simulink model "Mounir"  (R2015a)
settings: Solver=ode45  StartTime=0.0  StopTime=0.25  RelTol=1e-3
libraries: powerlib x31, simulink x4, powerlib_meascontrol x4, powerlib_extras x3
settings Model: Creator=USER  LastModifiedBy=USER
settings DebuggingCC: DiscreteInheritContinuousMsg=none

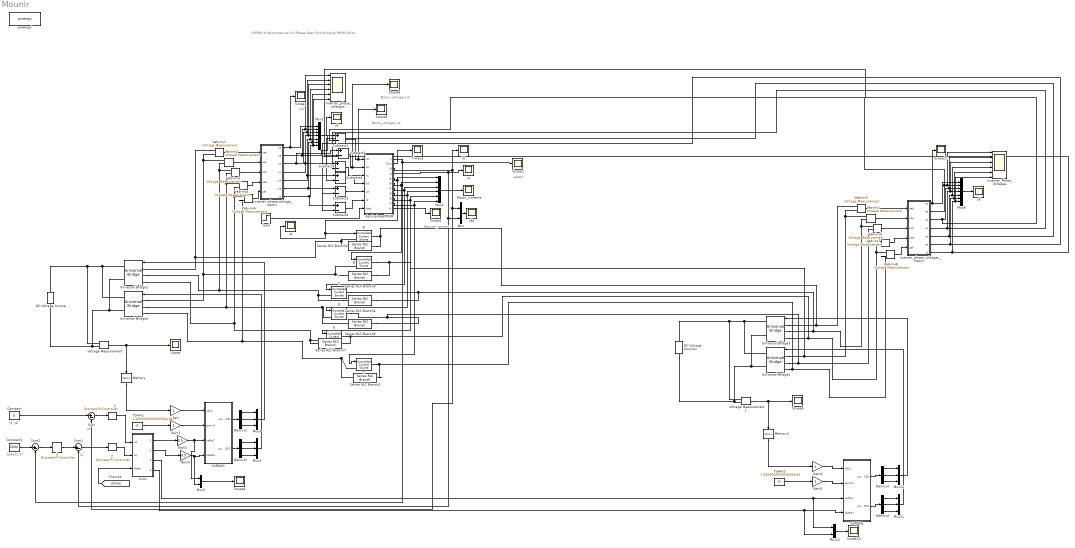
== system Mounir ==
  note: Neutral_current
  note: VSPWM of Asymmetrical Six Phase Open End Winding PMSM Drive
  note: Motor_voltage_Ub
  note: U0
  note: Motor_voltage_Ua
  note: speed
  note: Speed_ref
  note: Iq
  note: Id_ref
  note: Id
  "    1" : powerlib_extras/Discrete  Control Blocks/Discrete PI Controller  Kp=1  Ki=100  Par_Limits=[50 -50]  Init=0  Ts=1.000000000000000e-04
  " 1" : powerlib_extras/Discrete  Control Blocks/Discrete PI Controller  Kp=15  Ki=2000  Par_Limits=[300 -300]  Init=0  Ts=1.000000000000000e-04
  " 2" : powerlib_extras/Discrete  Control Blocks/Discrete PI Controller  Kp=15  Ki=2000  Par_Limits=[300 -300]  Init=0  Ts=1.000000000000000e-04
  2r/2s : Subsystem
  A : powerlib/Electrical Sources/Controlled Current Source  Initialize=on  Source_Type=AC  Amplitude=0  Phase=0  Frequency=0  Measurements=None
  B : powerlib/Electrical Sources/Controlled Current Source  Initialize=on  Source_Type=AC  Amplitude=0  Phase=0  Frequency=0  Measurements=None
  C : powerlib/Electrical Sources/Controlled Current Source  Initialize=on  Source_Type=AC  Amplitude=0  Phase=0  Frequency=0  Measurements=None
  Constant : Constant  Value=0
  Constant1 : Constant  Value=2000
  D : powerlib/Electrical Sources/Controlled Current Source  Initialize=on  Source_Type=AC  Amplitude=0  Phase=0  Frequency=0  Measurements=None
  DC Voltage Source : powerlib/Electrical Sources/DC Voltage Source  Amplitude=400  Measurements=None
  DC Voltage Source1 : powerlib/Electrical Sources/DC Voltage Source  Amplitude=400  Measurements=None
  Demux{1..4} (4 alike) : Demux  Outputs=3
  E : powerlib/Electrical Sources/Controlled Current Source  Initialize=on  Source_Type=AC  Amplitude=0  Phase=0  Frequency=0  Measurements=None
  F : powerlib/Electrical Sources/Controlled Current Source  Initialize=on  Source_Type=AC  Amplitude=0  Phase=0  Frequency=0  Measurements=None
  Gain{,1,4..5} (4 alike) : Gain  SampleTime=1.000000000000000e-04
  Gain2 : Gain  Gain=0.5  SampleTime=1.000000000000000e-04
  Gain3 : Gain  Gain=0.5  SampleTime=1.000000000000000e-04
  Inverter_Phase_Voltages : Scope  NumInputPorts=6
      settings: TimeRange=0.25  YMin=-400~-400~-400~-400~-400~-200  YMax=400~400~200~200~400~400  SaveName=ScopeData34
  Inverter_phase_volatges : Scope  NumInputPorts=6
      settings: TimeRange=0.25  YMin=-400~-400~-400~-400~-400~-200  YMax=400~400~200~200~400~400  SaveName=ScopeData10
  Memory : Memory
  Memory1 : Memory
  Motor_currents : Scope
      settings: TimeRange=0.162086856264412  YMin=-30  YMax=30  SaveName=ScopeData4
  Mux : Mux  Inputs=2
  Mux1 : Mux  Inputs=7
  Mux{3..4,10..11} (4 alike) : Mux  Inputs=3
  Mux12 : Mux  Inputs=2
  Mux2 : Mux  Inputs=6
  Mux5 : Mux  Inputs=2
  Mux8 : Mux  Inputs=7
  SVPWM1 : Subsystem
  SVPWM2 : Subsystem
  Scope{,1..2,4..6,8..11} (10 alike) : Scope
      Scope settings: YMin=487  YMax=501  SaveName=ScopeData7
      Scope1 settings: TimeRange=0.03905645784996133  YMin=2965  YMax=3002.5  SaveName=ScopeData15
      Scope10 settings: TimeRange=0.1492337164750958  YMin=-300  YMax=350  SaveName=ScopeData13
      Scope11 settings: TimeRange=0.05005764796310527  YMin=-2  YMax=2  SaveName=ScopeData14
      Scope2 settings: TimeRange=0.03905645784996133  YMin=2965  YMax=3002.5  SaveName=ScopeData2
      Scope4 settings: TimeRange=0.1492337164750958  YMin=-300  YMax=350  SaveName=ScopeData35
      Scope5 settings: TimeRange=0.05005764796310527  YMin=-2  YMax=2  SaveName=ScopeData5
      Scope6 settings: YMin=487  YMax=501  SaveName=ScopeData21
      Scope8 settings: TimeRange=0.05005764796310527  YMin=-2  YMax=2  SaveName=ScopeData30
      Scope9 settings: TimeRange=0.05005764796310527  YMin=-2  YMax=2  SaveName=ScopeData31
  Series RLC Branch{1..4,6..7} (6 alike) : powerlib/Elements/Series RLC Branch  LConnTagsString=__new0  RConnTagsString=__new0  BranchType=R  Resistance=10e10  Inductance=10e-7  SetiL0=off  InitialCurrent=0  Capacitance=1e-6  Setx0=off  InitialVoltage=0  Measurements=None
  Subtract{1..6} (6 alike) : Sum  Inputs=+-
  Sum : Sum  Inputs=|+-
  Sum1 : Sum  Inputs=|+-
  Sum2 : Sum  Inputs=|+-
  Torque : Scope
      settings: TimeRange=0.02996906419180202  YMin=-2  YMax=2  SaveName=ScopeData3
  Tpwm1 : Constant  Value=1.000000000000000e-04
  Tpwm2 : Constant  Value=1.000000000000000e-04
  Universal Bridge{1..4} (4 alike) : powerlib/Power Electronics/Universal Bridge  Arms=3  SnubberResistance=1e5  SnubberCapacitance=inf  Device=IGBT / Diodes  Ron=1e-3  Lon=0  ForwardVoltages="[  0  0  ]"  ForwardVoltage=0  GTOparameters=[ 10e-6 , 20e-6 ]  IGBTparameters=[ 1e-6 , 2e-6 ]  Measurements=None  Measurements_2=None  converterType=Rectifier
  Vab-inv{1..8} (8 alike) : powerlib/Measurements/Voltage Measurement  Tag=PoWeRsYsTeMmEaSuReMeNt  PhasorSimulation=off  OutputType=Magnitude  PSBequivalent=0
  Vbc-inv1 : powerlib/Measurements/Voltage Measurement  Tag=PoWeRsYsTeMmEaSuReMeNt  PhasorSimulation=off  OutputType=Magnitude  PSBequivalent=0
  Vbc-inv2 : powerlib/Measurements/Voltage Measurement  Tag=PoWeRsYsTeMmEaSuReMeNt  PhasorSimulation=off  OutputType=Magnitude  PSBequivalent=0
  Voltage Measurement : powerlib/Measurements/Voltage Measurement  PhasorSimulation=off  OutputType=Complex  PSBequivalent=0
  Voltage Measurement1 : powerlib/Measurements/Voltage Measurement  PhasorSimulation=off  OutputType=Complex  PSBequivalent=0
  dq-sixphasePMSM : Subsystem  mask{R=0.099, Ld=2.46068e-3, Lq=2.4759e-3, Lf=1.520747e-3, psi=0.0592, p=5, J=0.00174}
      mask prompts: R "Resistance (Om)"; Ld "d-inductance (H)"; Lq "q-inductance (H)"; Lf "Leak inductance (H)"; psi "flux (Wb)"; p "pole pairs"; J "inertia (kg*m^2)"
  iA : Scope
      settings: TimeRange=0.0250173024610546  YMin=-4  YMax=3.5  SaveName=ScopeData16
  id : Scope
      settings: YMin=-3  YMax=3
  idq : Scope
      settings: YMin=-20  YMax=50  SaveName=ScopeData12
  "inverter -phase-voltage_matrix " : MATLAB Function  TreatAsAtomicUnit=on
  inverter_phase_voltages_matrix : MATLAB Function  TreatAsAtomicUnit=on
  iq : Scope
      settings: TimeRange=0.01114527286702537  YMin=-4  YMax=4
  load : Step  Time=0  After=20  SampleTime=0
  powergui : powerlib/powergui  Priority=1  SimulationMode=Discrete  SolverType=Tustin  SampleTime=1e-6  frequency=60  SPID=off  DisableSnubberDevices=off  DisableRonSwitches=off  DisableVfSwitches=off  SwTol=0  DisplayEquations=off  Interpol=off  methode=off  Ts=0  FunctionMessages=off  echomessages=off  HookPort=off  EnableUseOfTLC=off  x0status=blocks  frequencyindice=0  Pbase=100e6  ErrMax=1e-4  Iterations=50  UnitsV=kV  UnitsW=MW  buscounter=0  RestoreLinks=warning  ResistiveCurrentMeasurement=off  Frange=[0:2:500]  Ylog=off  Xlog=on  ShowGrid=off  save=off  variable=ZData  structure=ScopeData16  ZoomFFT=off  StartTime=0.2  cycles=1  DisplayStyle=1  fundamental=50  FreqAxis=on  MaxFrequency=5000  frequencyindicesteady=1  RmsSteady=1  display=off
  u2 : Scope
      settings: TimeRange=0.25  YMin=-400  YMax=400  SaveName=ScopeData6
  u5 : Scope
      settings: TimeRange=0.25  YMin=-400  YMax=400  SaveName=ScopeData36
  wires:
  load/1 -> dq-sixphasePMSM/7(load)
  dq-sixphasePMSM/5(iA) -> Mux2/1, iA/1, A/1
  dq-sixphasePMSM/6(iB) -> Mux2/2, B/1
  dq-sixphasePMSM/7(iC) -> Mux2/3, C/1
  dq-sixphasePMSM/8(iD) -> Mux2/4, D/1
  dq-sixphasePMSM/9(iE) -> Mux2/5, E/1
  dq-sixphasePMSM/10(iF) -> Mux2/6, F/1
  Mux1/1 -> u2/1
  Vab-inv1/1 -> "inverter -phase-voltage_matrix "/1(uab)
  Vbc-inv2/1 -> "inverter -phase-voltage_matrix "/2(ubc)
  Vab-inv3/1 -> "inverter -phase-voltage_matrix "/3(ucd)
  Vab-inv4/1 -> "inverter -phase-voltage_matrix "/4(ude)
  Vab-inv6/1 -> "inverter -phase-voltage_matrix "/5(uef)
  "inverter -phase-voltage_matrix "/2(ua) -> Subtract1/1, Mux1/2, Inverter_phase_volatges/1
  "inverter -phase-voltage_matrix "/3(ub) -> Subtract2/1, Mux1/3, Inverter_phase_volatges/2
  "inverter -phase-voltage_matrix "/4(uc) -> Subtract3/1, Mux1/4, Inverter_phase_volatges/3
  "inverter -phase-voltage_matrix "/5(ud) -> Subtract4/1, Mux1/5, Inverter_phase_volatges/4
  "inverter -phase-voltage_matrix "/6(ue) -> Mux1/6, Inverter_phase_volatges/5, Subtract5/1
  "inverter -phase-voltage_matrix "/7(uf) -> Subtract6/1, Mux1/7, Inverter_phase_volatges/6
  "inverter -phase-voltage_matrix "/1(uo) -> Scope5/1, Mux1/1
  Mux/1 -> idq/1
  dq-sixphasePMSM/1(n) -> Sum2/2, Scope2/1
  dq-sixphasePMSM/3(id) -> Sum/2, Mux/1, id/1
  dq-sixphasePMSM/4(iq) -> Sum1/2, Mux/2, iq/1
  Tpwm1/1 -> Gain1/1
  Sum1/1 -> " 2"/1
  Constant/1 -> Sum/1
  Sum2/1 -> "    1"/1
  Constant1/1 -> Sum2/1
  [phase] -> 2r/2s/3(theta)
  Mux3/1 -> Universal Bridge1/1
  Demux1/2 -> Mux3/2
  Mux5/1 -> Scope4/1
  Memory/1 -> Gain/1
  Mux4/1 -> Universal Bridge2/1
  Mux2/1 -> Motor_currents/1
  "    1"/1 -> Sum1/1
  Sum/1 -> " 1"/1
  " 1"/1 -> 2r/2s/1(ud)
  " 2"/1 -> 2r/2s/2(uq)
  Demux2/2 -> Mux4/2
  Demux2/1 -> Mux4/1
  Demux1/1 -> Mux3/1
  Demux1/3 -> Mux3/3
  Demux2/3 -> Mux4/3
  Voltage Measurement/1 -> Memory/1, Scope/1
  Gain/1 -> SVPWM1/1(udc1)
  Gain1/1 -> SVPWM1/2(tpwm1)
  Gain2/1 -> Mux5/1, SVPWM1/3(ualfa1)
  Gain3/1 -> Mux5/2, SVPWM1/4(ubeta1)
  SVPWM1/1(pwm_ACE1) -> Demux1/1
  SVPWM1/2(pwm_BDF1) -> Demux2/1
  Mux8/1 -> u5/1
  Vab-inv2/1 -> inverter_phase_voltages_matrix/1(uab)
  Vbc-inv1/1 -> inverter_phase_voltages_matrix/2(ubc)
  Vab-inv5/1 -> inverter_phase_voltages_matrix/3(ucd)
  Vab-inv7/1 -> inverter_phase_voltages_matrix/4(ude)
  Vab-inv8/1 -> inverter_phase_voltages_matrix/5(uef)
  inverter_phase_voltages_matrix/2(ua) -> Subtract1/2, Mux8/2, Inverter_Phase_Voltages/1
  inverter_phase_voltages_matrix/3(ub) -> Subtract2/2, Mux8/3, Inverter_Phase_Voltages/2
  inverter_phase_voltages_matrix/4(uc) -> Subtract3/2, Mux8/4, Inverter_Phase_Voltages/3
  inverter_phase_voltages_matrix/5(ud) -> Subtract4/2, Mux8/5, Inverter_Phase_Voltages/4
  inverter_phase_voltages_matrix/6(ue) -> Subtract5/2, Mux8/6, Inverter_Phase_Voltages/5
  inverter_phase_voltages_matrix/7(uf) -> Subtract6/2, Mux8/7, Inverter_Phase_Voltages/6
  inverter_phase_voltages_matrix/1(uo) -> Scope11/1, Mux8/1
  Tpwm2/1 -> Gain5/1
  Demux3/2 -> Mux10/2
  Mux12/1 -> Scope10/1
  Memory1/1 -> Gain4/1
  Mux11/1 -> Universal Bridge4/1
  2r/2s/4(ubeta2) -> SVPWM2/4(ubeta1), Mux12/2
  Demux4/2 -> Mux11/2
  Demux4/1 -> Mux11/1
  Demux3/1 -> Mux10/1
  Demux3/3 -> Mux10/3
  Demux4/3 -> Mux11/3
  Voltage Measurement1/1 -> Memory1/1, Scope6/1
  Gain4/1 -> SVPWM2/1(udc1)
  Gain5/1 -> SVPWM2/2(tpwm1)
  2r/2s/3(ualfa2) -> Mux12/1, SVPWM2/3(ualfa1)
  SVPWM2/1(pwm_ACE1) -> Demux3/1
  SVPWM2/2(pwm_BDF1) -> Demux4/1
  Mux10/1 -> Universal Bridge3/1
  2r/2s/1(ualfa1) -> Gain2/1
  2r/2s/2(ubeta1) -> Gain3/1
  Subtract1/1 -> Scope9/1, dq-sixphasePMSM/1(ua)
  Subtract2/1 -> dq-sixphasePMSM/2(ub), Scope8/1
  Subtract3/1 -> dq-sixphasePMSM/3(uc)
  Subtract4/1 -> dq-sixphasePMSM/4(ud)
  Subtract5/1 -> dq-sixphasePMSM/5(ue)
  Subtract6/1 -> dq-sixphasePMSM/6(uf)
  dq-sixphasePMSM/2(Tem) -> Torque/1
  dq-sixphasePMSM/11(In) -> Scope1/1
  connections:
  Vab-inv1/LConn1 -- Universal Bridge1/LConn1 -- A/LConn1 -- Series RLC Branch2/LConn1
  Series RLC Branch3/LConn1 -- B/LConn1 -- Universal Bridge2/LConn1 -- Vbc-inv2/LConn1 -- Vab-inv1/LConn2
  Series RLC Branch4/LConn1 -- C/LConn1 -- Universal Bridge1/LConn2 -- Vbc-inv2/LConn2 -- Vab-inv3/LConn1
  Universal Bridge2/LConn2 -- Series RLC Branch6/LConn1 -- D/LConn1 -- Vab-inv4/LConn1 -- Vab-inv3/LConn2
  Series RLC Branch7/LConn1 -- E/LConn1 -- Universal Bridge1/LConn3 -- Vab-inv4/LConn2 -- Vab-inv6/LConn1
  Vab-inv6/LConn2 -- Universal Bridge2/LConn3 -- Series RLC Branch1/LConn1 -- F/LConn1
  Universal Bridge2/RConn1 -- Universal Bridge1/RConn1 -- Voltage Measurement/LConn1 -- DC Voltage Source/RConn1
  Universal Bridge1/RConn2 -- Universal Bridge2/RConn2 -- Voltage Measurement/LConn2 -- DC Voltage Source/LConn1
  Vab-inv2/LConn1 -- Universal Bridge3/LConn1 -- Series RLC Branch2/RConn1 -- A/RConn1
  Vab-inv2/LConn2 -- Vbc-inv1/LConn1 -- Series RLC Branch3/RConn1 -- B/RConn1 -- Universal Bridge4/LConn1
  Vab-inv5/LConn2 -- Vab-inv7/LConn1 -- D/RConn1 -- Series RLC Branch6/RConn1 -- Universal Bridge4/LConn2
  Vab-inv8/LConn2 -- Universal Bridge4/LConn3 -- Series RLC Branch1/RConn1 -- F/RConn1
  Universal Bridge4/RConn1 -- Universal Bridge3/RConn1 -- DC Voltage Source1/RConn1 -- Voltage Measurement1/LConn1
  Universal Bridge3/RConn2 -- Universal Bridge4/RConn2 -- DC Voltage Source1/LConn1 -- Voltage Measurement1/LConn2
  Vab-inv5/LConn1 -- Vbc-inv1/LConn2 -- Universal Bridge3/LConn2 -- C/RConn1 -- Series RLC Branch4/RConn1
  Vab-inv8/LConn1 -- Vab-inv7/LConn2 -- Universal Bridge3/LConn3 -- Series RLC Branch7/RConn1 -- E/RConn1

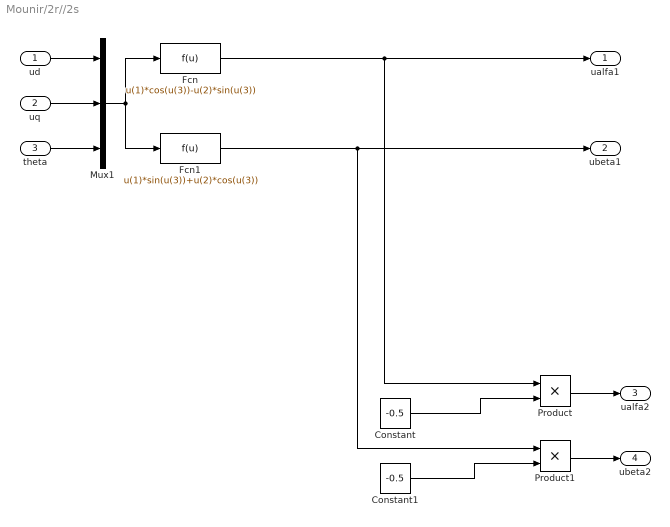
== system Mounir/2r//2s ==
  ud : Inport
  uq : Inport  Port=2
  theta : Inport  Port=3
  Constant : Constant  Value=-0.5
  Constant1 : Constant  Value=-0.5
  Fcn : Fcn  Expr=u(1)*cos(u(3))-u(2)*sin(u(3))
  Fcn1 : Fcn  Expr=u(1)*sin(u(3))+u(2)*cos(u(3))
  Mux1 : Mux  Inputs=3
  Product : Product
  Product1 : Product
  ualfa1 : Outport
  ubeta1 : Outport  Port=2
  ualfa2 : Outport  Port=3
  ubeta2 : Outport  Port=4
  wires:
  theta/1 -> Mux1/3
  uq/1 -> Mux1/2
  ud/1 -> Mux1/1
  Mux1/1 -> Fcn1/1, Fcn/1
  Fcn/1 -> Product/1, ualfa1/1
  Fcn1/1 -> Product1/1, ubeta1/1
  Constant/1 -> Product/2
  Product1/1 -> ubeta2/1
  Product/1 -> ualfa2/1
  Constant1/1 -> Product1/2

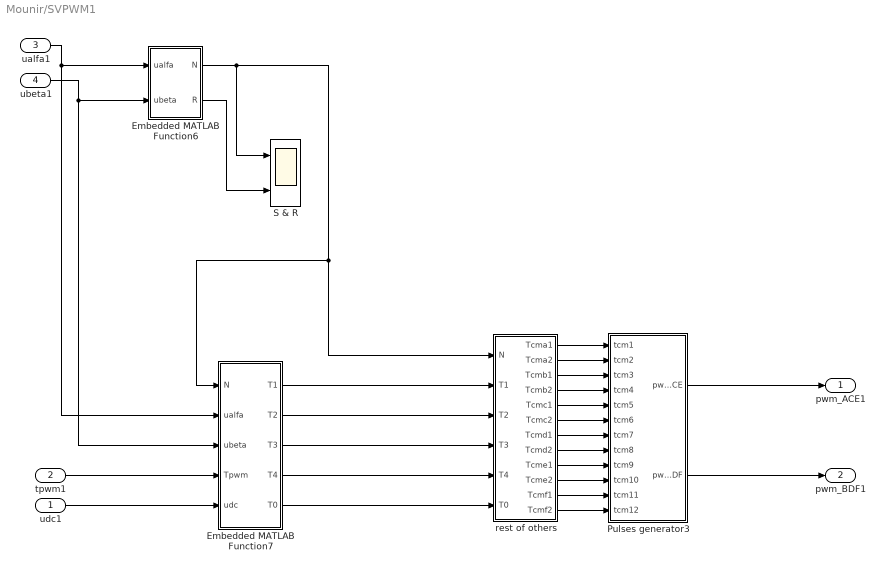
== system Mounir/SVPWM1 ==
  udc1 : Inport
  tpwm1 : Inport  Port=2
  ualfa1 : Inport  Port=3
  ubeta1 : Inport  Port=4
  Embedded MATLAB Function6 : MATLAB Function  TreatAsAtomicUnit=on
  Embedded MATLAB Function7 : MATLAB Function  TreatAsAtomicUnit=on
  Pulses generator3 : Subsystem
  S & R : Scope  NumInputPorts=2
      settings: TimeRange=0.00012  YMin=-1~-1  YMax=2~2  SaveName=ScopeData40
  rest of others : MATLAB Function  TreatAsAtomicUnit=on
  pwm_ACE1 : Outport
  pwm_BDF1 : Outport  Port=2
  wires:
  ualfa1/1 -> Embedded MATLAB Function7/2(ualfa), Embedded MATLAB Function6/1(ualfa)
  ubeta1/1 -> Embedded MATLAB Function7/3(ubeta), Embedded MATLAB Function6/2(ubeta)
  Pulses generator3/2(pwm_BDF) -> pwm_BDF1/1
  Pulses generator3/1(pwm_ACE) -> pwm_ACE1/1
  tpwm1/1 -> Embedded MATLAB Function7/4(Tpwm)
  udc1/1 -> Embedded MATLAB Function7/5(udc)
  Embedded MATLAB Function7/1(T1) -> rest of others/2(T1)
  Embedded MATLAB Function7/2(T2) -> rest of others/3(T2)
  Embedded MATLAB Function7/3(T3) -> rest of others/4(T3)
  Embedded MATLAB Function7/4(T4) -> rest of others/5(T4)
  Embedded MATLAB Function7/5(T0) -> rest of others/6(T0)
  Embedded MATLAB Function6/1(N) -> S & R/1, rest of others/1(N), Embedded MATLAB Function7/1(N)
  rest of others/3(Tcmb1) -> Pulses generator3/3(tcm3)
  rest of others/2(Tcma2) -> Pulses generator3/2(tcm2)
  rest of others/8(Tcmd2) -> Pulses generator3/8(tcm8)
  rest of others/4(Tcmb2) -> Pulses generator3/4(tcm4)
  rest of others/5(Tcmc1) -> Pulses generator3/5(tcm5)
  rest of others/9(Tcme1) -> Pulses generator3/9(tcm9)
  rest of others/1(Tcma1) -> Pulses generator3/1(tcm1)
  rest of others/10(Tcme2) -> Pulses generator3/10(tcm10)
  rest of others/6(Tcmc2) -> Pulses generator3/6(tcm6)
  rest of others/7(Tcmd1) -> Pulses generator3/7(tcm7)
  rest of others/11(Tcmf1) -> Pulses generator3/11(tcm11)
  rest of others/12(Tcmf2) -> Pulses generator3/12(tcm12)
  Embedded MATLAB Function6/2(R) -> S & R/2

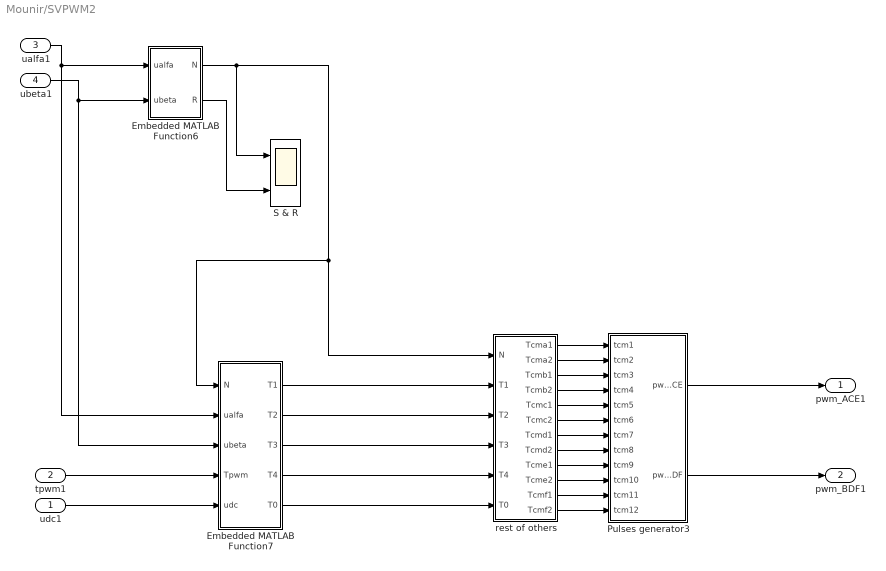
== system Mounir/SVPWM2 ==
  udc1 : Inport
  tpwm1 : Inport  Port=2
  ualfa1 : Inport  Port=3
  ubeta1 : Inport  Port=4
  Embedded MATLAB Function6 : MATLAB Function  TreatAsAtomicUnit=on
  Embedded MATLAB Function7 : MATLAB Function  TreatAsAtomicUnit=on
  Pulses generator3 : Subsystem
  S & R : Scope  NumInputPorts=2
      settings: TimeRange=0.00012  YMin=-1~-1  YMax=2~2  SaveName=ScopeData40
  rest of others : MATLAB Function  TreatAsAtomicUnit=on
  pwm_ACE1 : Outport
  pwm_BDF1 : Outport  Port=2
  wires:
  ualfa1/1 -> Embedded MATLAB Function7/2(ualfa), Embedded MATLAB Function6/1(ualfa)
  ubeta1/1 -> Embedded MATLAB Function7/3(ubeta), Embedded MATLAB Function6/2(ubeta)
  Pulses generator3/2(pwm_BDF) -> pwm_BDF1/1
  Pulses generator3/1(pwm_ACE) -> pwm_ACE1/1
  tpwm1/1 -> Embedded MATLAB Function7/4(Tpwm)
  udc1/1 -> Embedded MATLAB Function7/5(udc)
  Embedded MATLAB Function7/1(T1) -> rest of others/2(T1)
  Embedded MATLAB Function7/2(T2) -> rest of others/3(T2)
  Embedded MATLAB Function7/3(T3) -> rest of others/4(T3)
  Embedded MATLAB Function7/4(T4) -> rest of others/5(T4)
  Embedded MATLAB Function7/5(T0) -> rest of others/6(T0)
  Embedded MATLAB Function6/1(N) -> S & R/1, rest of others/1(N), Embedded MATLAB Function7/1(N)
  rest of others/3(Tcmb1) -> Pulses generator3/3(tcm3)
  rest of others/2(Tcma2) -> Pulses generator3/2(tcm2)
  rest of others/8(Tcmd2) -> Pulses generator3/8(tcm8)
  rest of others/4(Tcmb2) -> Pulses generator3/4(tcm4)
  rest of others/5(Tcmc1) -> Pulses generator3/5(tcm5)
  rest of others/9(Tcme1) -> Pulses generator3/9(tcm9)
  rest of others/1(Tcma1) -> Pulses generator3/1(tcm1)
  rest of others/10(Tcme2) -> Pulses generator3/10(tcm10)
  rest of others/6(Tcmc2) -> Pulses generator3/6(tcm6)
  rest of others/7(Tcmd1) -> Pulses generator3/7(tcm7)
  rest of others/11(Tcmf1) -> Pulses generator3/11(tcm11)
  rest of others/12(Tcmf2) -> Pulses generator3/12(tcm12)
  Embedded MATLAB Function6/2(R) -> S & R/2

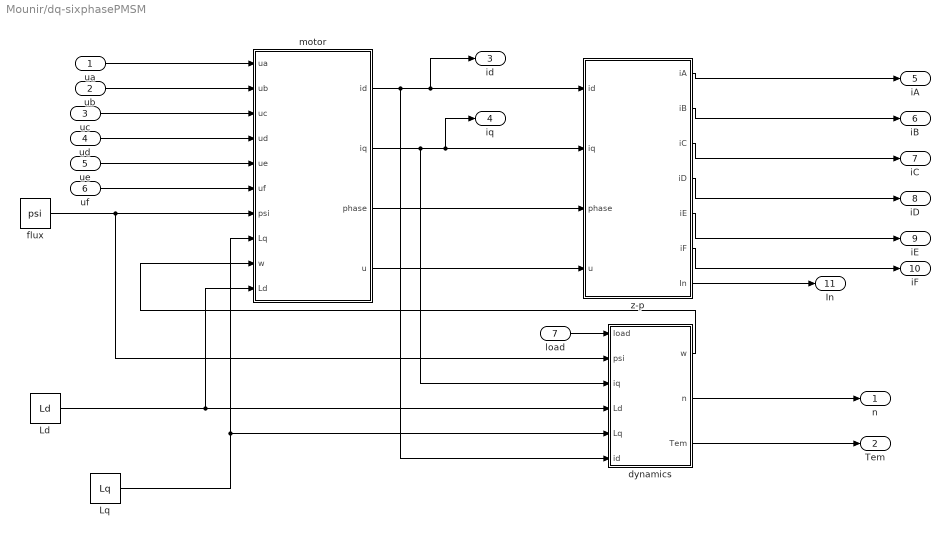
== system Mounir/dq-sixphasePMSM ==
  ua : Inport
  ub : Inport  Port=2
  uc : Inport  Port=3
  ud : Inport  Port=4
  ue : Inport  Port=5
  uf : Inport  Port=6
  load : Inport  Port=7
  Ld : Constant  Value=Ld
  Lq : Constant  Value=Lq
  dynamics : Subsystem
  flux : Constant  Value=psi
  motor : Subsystem
  z-p : Subsystem
  n : Outport
  Tem : Outport  Port=2
  id : Outport  Port=3
  iq : Outport  Port=4
  iA : Outport  Port=5
  iB : Outport  Port=6
  iC : Outport  Port=7
  iD : Outport  Port=8
  iE : Outport  Port=9
  iF : Outport  Port=10
  In : Outport  Port=11
  wires:
  Lq/1 -> motor/8(Lq), dynamics/5(Lq)
  Ld/1 -> dynamics/4(Ld), motor/10(Ld)
  ud/1 -> motor/4(ud)
  ua/1 -> motor/1(ua)
  ue/1 -> motor/5(ue)
  ub/1 -> motor/2(ub)
  uf/1 -> motor/6(uf)
  uc/1 -> motor/3(uc)
  dynamics/2(n) -> n/1
  load/1 -> dynamics/1(load)
  z-p/1(iA) -> iA/1
  motor/1(id) -> dynamics/6(id), z-p/1(id), id/1
  motor/2(iq) -> dynamics/3(iq), z-p/2(iq), iq/1
  motor/4(u) -> z-p/4(u)
  dynamics/1(w) -> motor/9(w)
  dynamics/3(Tem) -> Tem/1
  flux/1 -> dynamics/2(psi), motor/7(psi)
  z-p/2(iB) -> iB/1
  z-p/3(iC) -> iC/1
  z-p/4(iD) -> iD/1
  z-p/5(iE) -> iE/1
  z-p/6(iF) -> iF/1
  motor/3(phase) -> z-p/3(phase)
  z-p/7(In) -> In/1

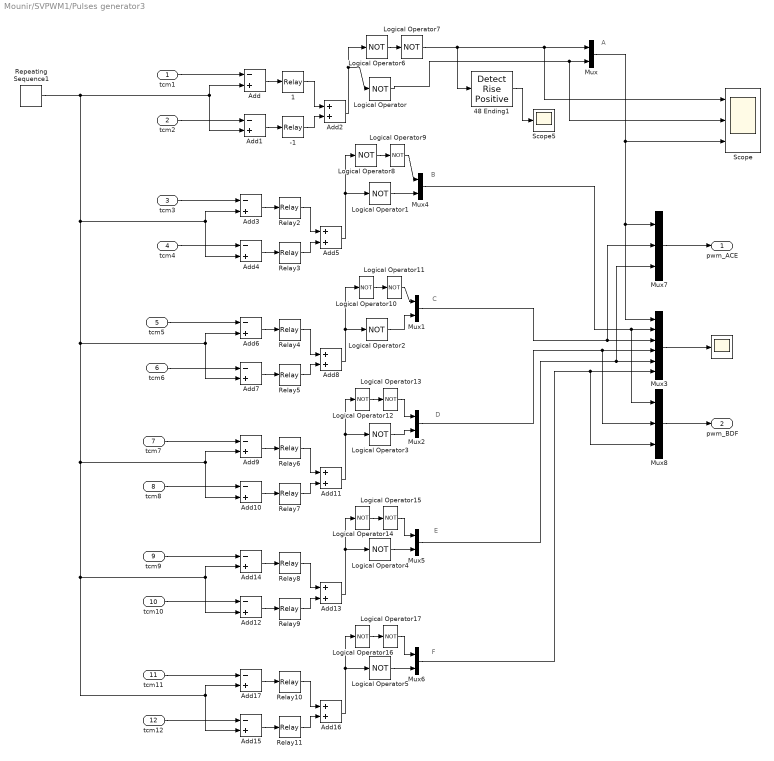
== system Mounir/SVPWM1/Pulses generator3 ==
  note: F
  note: E
  note: D
  note: C
  note: B
  note: A
  tcm1 : Inport
  tcm2 : Inport  Port=2
  tcm3 : Inport  Port=3
  tcm4 : Inport  Port=4
  tcm5 : Inport  Port=5
  tcm6 : Inport  Port=6
  tcm7 : Inport  Port=7
  tcm8 : Inport  Port=8
  tcm9 : Inport  Port=9
  tcm10 : Inport  Port=10
  tcm11 : Inport  Port=11
  tcm12 : Inport  Port=12
  " " : Scope
      settings: TimeRange=0.07697852690247936  YMin=-15  YMax=15  SaveName=ScopeData27
  -1 : Relay  OnOutputValue=-1
  1 : Relay
  48 Ending1 : simulink/Logic and Bit Operations/Detect Rise Positive  vinit=0  InputProcessing=Inherited  OutDataTypeStr=boolean
  Add{,1,3..4,6..7,9..10,12,14..15,17} (12 alike) : Sum  Inputs=-+
  Add{2,5,8,11,13,16} (6 alike) : Sum
  Logical Operator{,1..17} (18 alike) : Logic  Operator=NOT  AllPortsSameDT=off  OutDataTypeStr=boolean
  Mux{,1..2,4..6} (6 alike) : Mux  Inputs=2
  Mux3 : Mux  Inputs=6
  Mux7 : Mux  Inputs=3
  Mux8 : Mux  Inputs=3
  Relay{2,4,6,8,10} (5 alike) : Relay
  Relay{3,5,7,9,11} (5 alike) : Relay  OnOutputValue=-1
  Repeating Sequence1 : simulink/Sources/Repeating Sequence  rep_seq_t=[0 1.000000000000000e-04]  rep_seq_y=[0 1.000000000000000e-04]
  Scope : Scope  NumInputPorts=3
      settings: YMin=-5~-5~-5  YMax=5~5~5  SaveName=ScopeData22
  Scope5 : Scope
      settings: TimeRange=0.05005764796310527  YMin=-2  YMax=2  SaveName=ScopeData26
  pwm_ACE : Outport
  pwm_BDF : Outport  Port=2
  wires:
  Mux6/1 -> Mux8/3, Mux3/6
  Mux5/1 -> Mux7/3, Mux3/5
  Mux2/1 -> Mux8/2, Mux3/4
  Mux1/1 -> Mux7/2, Mux3/3
  Mux4/1 -> Mux8/1, Mux3/2
  tcm5/1 -> Add6/1
  tcm3/1 -> Add3/1
  tcm2/1 -> Add1/1
  Repeating Sequence1/1 -> Add/2, Add1/2, Add4/2, Add3/2, Add6/2, Add7/2, Add10/2, Add9/2, Add14/2, Add12/2, Add15/2, Add17/2
  Add/1 -> 1/1
  Add1/1 -> -1/1
  1/1 -> Add2/1
  -1/1 -> Add2/2
  tcm1/1 -> Add/1
  Add2/1 -> Logical Operator6/1, Logical Operator/1
  Logical Operator1/1 -> Mux4/2
  Add3/1 -> Relay2/1
  Add4/1 -> Relay3/1
  Relay2/1 -> Add5/1
  Relay3/1 -> Add5/2
  Add5/1 -> Logical Operator1/1, Logical Operator8/1
  tcm4/1 -> Add4/1
  Logical Operator2/1 -> Mux1/2
  Add6/1 -> Relay4/1
  Add7/1 -> Relay5/1
  Relay4/1 -> Add8/1
  Relay5/1 -> Add8/2
  Add8/1 -> Logical Operator10/1, Logical Operator2/1
  tcm6/1 -> Add7/1
  tcm7/1 -> Add9/1
  Logical Operator3/1 -> Mux2/2
  Add9/1 -> Relay6/1
  Add10/1 -> Relay7/1
  Relay6/1 -> Add11/1
  Relay7/1 -> Add11/2
  Add11/1 -> Logical Operator3/1, Logical Operator12/1
  tcm8/1 -> Add10/1
  tcm9/1 -> Add14/1
  Add14/1 -> Relay8/1
  Add12/1 -> Relay9/1
  Relay8/1 -> Add13/1
  Relay9/1 -> Add13/2
  Add13/1 -> Logical Operator4/1, Logical Operator14/1
  tcm10/1 -> Add12/1
  Logical Operator4/1 -> Mux5/2
  tcm11/1 -> Add17/1
  Add17/1 -> Relay10/1
  Add15/1 -> Relay11/1
  Relay10/1 -> Add16/1
  Relay11/1 -> Add16/2
  Add16/1 -> Logical Operator5/1, Logical Operator16/1
  tcm12/1 -> Add15/1
  Logical Operator5/1 -> Mux6/2
  Logical Operator6/1 -> Logical Operator7/1
  Logical Operator8/1 -> Logical Operator9/1
  Logical Operator9/1 -> Mux4/1
  Logical Operator10/1 -> Logical Operator11/1
  Logical Operator11/1 -> Mux1/1
  Logical Operator12/1 -> Logical Operator13/1
  Logical Operator13/1 -> Mux2/1
  Logical Operator14/1 -> Logical Operator15/1
  Logical Operator15/1 -> Mux5/1
  Logical Operator16/1 -> Logical Operator17/1
  Logical Operator17/1 -> Mux6/1
  Logical Operator/1 -> Scope/2, Mux/2
  Logical Operator7/1 -> 48 Ending1/1, Scope/1, Mux/1
  Mux/1 -> Mux7/1, Mux3/1, Scope/3
  Mux7/1 -> pwm_ACE/1
  Mux8/1 -> pwm_BDF/1
  48 Ending1/1 -> Scope5/1
  Mux3/1 -> " "/1

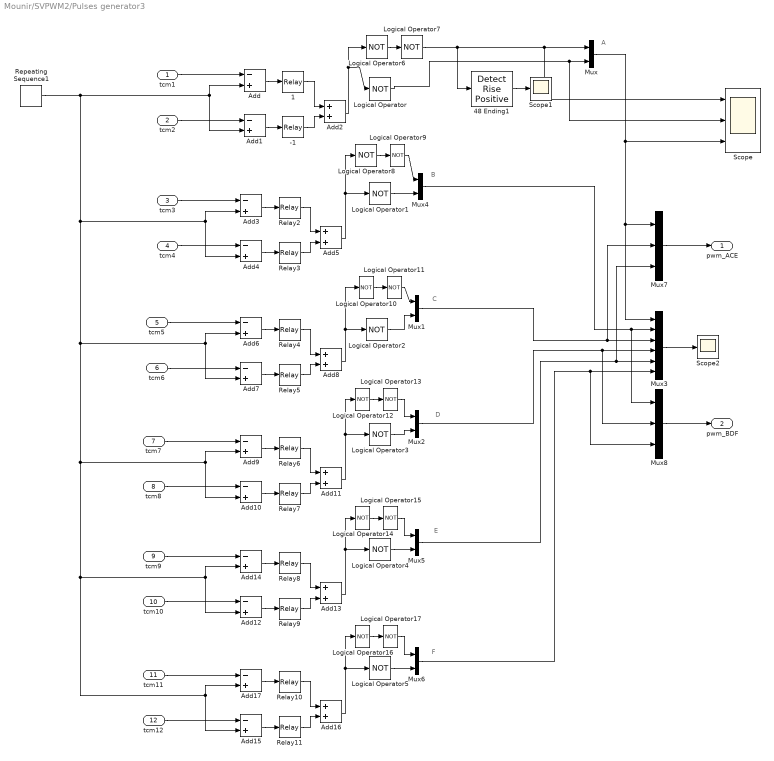
== system Mounir/SVPWM2/Pulses generator3 ==
  note: F
  note: E
  note: D
  note: C
  note: B
  note: A
  tcm1 : Inport
  tcm2 : Inport  Port=2
  tcm3 : Inport  Port=3
  tcm4 : Inport  Port=4
  tcm5 : Inport  Port=5
  tcm6 : Inport  Port=6
  tcm7 : Inport  Port=7
  tcm8 : Inport  Port=8
  tcm9 : Inport  Port=9
  tcm10 : Inport  Port=10
  tcm11 : Inport  Port=11
  tcm12 : Inport  Port=12
  -1 : Relay  OnOutputValue=-1
  1 : Relay
  48 Ending1 : simulink/Logic and Bit Operations/Detect Rise Positive  vinit=0  InputProcessing=Inherited  OutDataTypeStr=boolean
  Add{,1,3..4,6..7,9..10,12,14..15,17} (12 alike) : Sum  Inputs=-+
  Add{2,5,8,11,13,16} (6 alike) : Sum
  Logical Operator{,1..17} (18 alike) : Logic  Operator=NOT  AllPortsSameDT=off  OutDataTypeStr=boolean
  Mux{,1..2,4..6} (6 alike) : Mux  Inputs=2
  Mux3 : Mux  Inputs=6
  Mux7 : Mux  Inputs=3
  Mux8 : Mux  Inputs=3
  Relay{2,4,6,8,10} (5 alike) : Relay
  Relay{3,5,7,9,11} (5 alike) : Relay  OnOutputValue=-1
  Repeating Sequence1 : simulink/Sources/Repeating Sequence  rep_seq_t=[0 1.000000000000000e-04]  rep_seq_y=[0 1.000000000000000e-04]
  Scope : Scope  NumInputPorts=3
      settings: YMin=-5~-5~-5  YMax=5~5~5  SaveName=ScopeData22
  Scope1 : Scope
      settings: YMin=537.15  YMax=537.75  SaveName=ScopeData28
  Scope2 : Scope
      settings: YMin=537.15  YMax=537.75  SaveName=ScopeData29
  pwm_ACE : Outport
  pwm_BDF : Outport  Port=2
  wires:
  Mux6/1 -> Mux8/3, Mux3/6
  Mux5/1 -> Mux7/3, Mux3/5
  Mux2/1 -> Mux8/2, Mux3/4
  Mux1/1 -> Mux7/2, Mux3/3
  Mux4/1 -> Mux8/1, Mux3/2
  tcm5/1 -> Add6/1
  tcm3/1 -> Add3/1
  tcm2/1 -> Add1/1
  Repeating Sequence1/1 -> Add/2, Add1/2, Add4/2, Add3/2, Add6/2, Add7/2, Add10/2, Add9/2, Add14/2, Add12/2, Add15/2, Add17/2
  Add/1 -> 1/1
  Add1/1 -> -1/1
  1/1 -> Add2/1
  -1/1 -> Add2/2
  tcm1/1 -> Add/1
  Add2/1 -> Logical Operator6/1, Logical Operator/1
  Logical Operator1/1 -> Mux4/2
  Add3/1 -> Relay2/1
  Add4/1 -> Relay3/1
  Relay2/1 -> Add5/1
  Relay3/1 -> Add5/2
  Add5/1 -> Logical Operator1/1, Logical Operator8/1
  tcm4/1 -> Add4/1
  Logical Operator2/1 -> Mux1/2
  Add6/1 -> Relay4/1
  Add7/1 -> Relay5/1
  Relay4/1 -> Add8/1
  Relay5/1 -> Add8/2
  Add8/1 -> Logical Operator10/1, Logical Operator2/1
  tcm6/1 -> Add7/1
  tcm7/1 -> Add9/1
  Logical Operator3/1 -> Mux2/2
  Add9/1 -> Relay6/1
  Add10/1 -> Relay7/1
  Relay6/1 -> Add11/1
  Relay7/1 -> Add11/2
  Add11/1 -> Logical Operator3/1, Logical Operator12/1
  tcm8/1 -> Add10/1
  tcm9/1 -> Add14/1
  Add14/1 -> Relay8/1
  Add12/1 -> Relay9/1
  Relay8/1 -> Add13/1
  Relay9/1 -> Add13/2
  Add13/1 -> Logical Operator4/1, Logical Operator14/1
  tcm10/1 -> Add12/1
  Logical Operator4/1 -> Mux5/2
  tcm11/1 -> Add17/1
  Add17/1 -> Relay10/1
  Add15/1 -> Relay11/1
  Relay10/1 -> Add16/1
  Relay11/1 -> Add16/2
  Add16/1 -> Logical Operator5/1, Logical Operator16/1
  tcm12/1 -> Add15/1
  Logical Operator5/1 -> Mux6/2
  Logical Operator6/1 -> Logical Operator7/1
  Logical Operator8/1 -> Logical Operator9/1
  Logical Operator9/1 -> Mux4/1
  Logical Operator10/1 -> Logical Operator11/1
  Logical Operator11/1 -> Mux1/1
  Logical Operator12/1 -> Logical Operator13/1
  Logical Operator13/1 -> Mux2/1
  Logical Operator14/1 -> Logical Operator15/1
  Logical Operator15/1 -> Mux5/1
  Logical Operator16/1 -> Logical Operator17/1
  Logical Operator17/1 -> Mux6/1
  Logical Operator/1 -> Scope/2, Mux/2
  Logical Operator7/1 -> 48 Ending1/1, Scope/1, Mux/1
  Mux/1 -> Mux7/1, Mux3/1, Scope/3
  Mux7/1 -> pwm_ACE/1
  Mux8/1 -> pwm_BDF/1
  48 Ending1/1 -> Scope1/1
  Mux3/1 -> Scope2/1

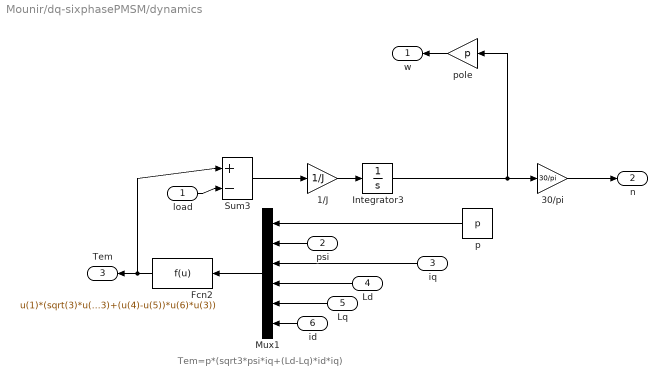
== system Mounir/dq-sixphasePMSM/dynamics ==
  note: Tem=p*(sqrt3*psi*iq+(Ld-Lq)*id*iq)
  load : Inport
  psi : Inport  Port=2
  iq : Inport  Port=3
  Ld : Inport  Port=4
  Lq : Inport  Port=5
  id : Inport  Port=6
  1/J : Gain  Gain=1/J  SaturateOnIntegerOverflow=on  OutDataTypeStr=Inherit: Same as input  ParamDataTypeStr=Inherit: Same as input
  30/pi : Gain  Gain=30/pi  SaturateOnIntegerOverflow=on  OutDataTypeStr=Inherit: Same as input  ParamDataTypeStr=Inherit: Same as input
  Fcn2 : Fcn  Expr=u(1)*(sqrt(3)*u(2)*u(3)+(u(4)-u(5))*u(6)*u(3))
  Integrator3 : Integrator
  Mux1 : Mux  Inputs=6
  Sum3 : Sum  Inputs=|+-  SaturateOnIntegerOverflow=on
  p : Constant  Value=p
  pole : Gain  Gain=p  SaturateOnIntegerOverflow=on  OutDataTypeStr=Inherit: Same as input  ParamDataTypeStr=Inherit: Same as input
  w : Outport
  n : Outport  Port=2
  Tem : Outport  Port=3
  wires:
  p/1 -> Mux1/1
  Mux1/1 -> Fcn2/1
  Fcn2/1 -> Sum3/1, Tem/1
  Sum3/1 -> 1/J/1
  1/J/1 -> Integrator3/1
  Integrator3/1 -> 30/pi/1, pole/1
  psi/1 -> Mux1/2
  Ld/1 -> Mux1/4
  Lq/1 -> Mux1/5
  pole/1 -> w/1
  30/pi/1 -> n/1
  load/1 -> Sum3/2
  iq/1 -> Mux1/3
  id/1 -> Mux1/6

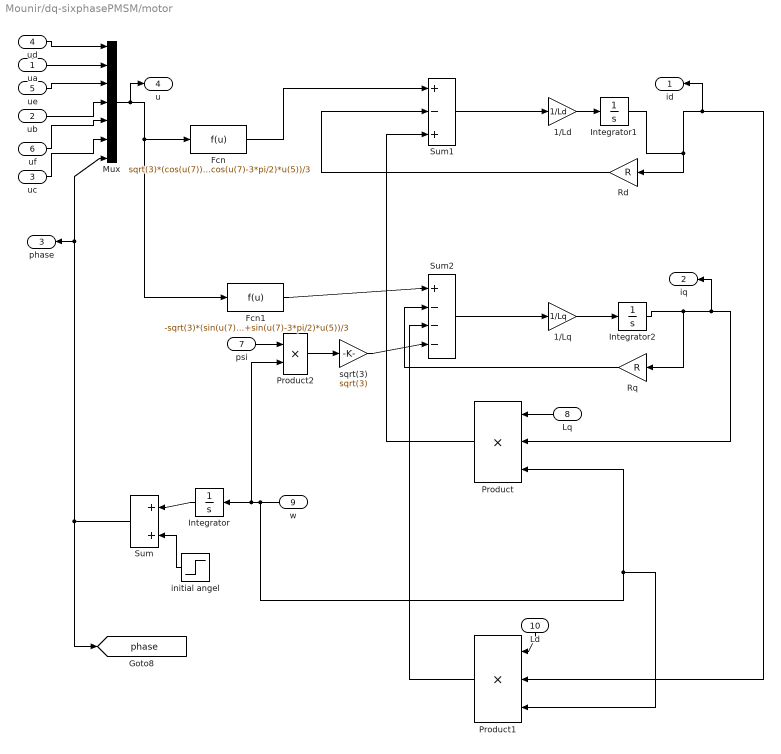
== system Mounir/dq-sixphasePMSM/motor ==
  ua : Inport
  ub : Inport  Port=2
  uc : Inport  Port=3
  ud : Inport  Port=4
  ue : Inport  Port=5
  uf : Inport  Port=6
  psi : Inport  Port=7
  Lq : Inport  Port=8
  w : Inport  Port=9
  Ld : Inport  Port=10
  1/Ld : Gain  Gain=1/Ld  SaturateOnIntegerOverflow=on  OutDataTypeStr=Inherit: Same as input  ParamDataTypeStr=Inherit: Same as input
  1/Lq : Gain  Gain=1/Lq  SaturateOnIntegerOverflow=on  OutDataTypeStr=Inherit: Same as input  ParamDataTypeStr=Inherit: Same as input
  Fcn : Fcn  Expr=sqrt(3)*(cos(u(7))*u(2)+cos(u(7)-pi/6)*u(4)+cos(u(7)-2*pi/3)*u(6)+cos(u(7)-5*pi/6)*u(1)+cos(u(7)-4*pi/3)*u(3)+cos(u(7)-3*pi/2)*u(5))/3
  Fcn1 : Fcn  Expr=-sqrt(3)*(sin(u(7))*u(2)+sin(u(7)-pi/6)*u(4)+sin(u(7)-2*pi/3)*u(6)+sin(u(7)-5*pi/6)*u(1)+sin(u(7)-4*pi/3)*u(3)+sin(u(7)-3*pi/2)*u(5))/3
  Integrator : Integrator
  Integrator1 : Integrator
  Integrator2 : Integrator
  Mux : Mux  Inputs=7
  Product : Product  Inputs=3  SaturateOnIntegerOverflow=on  OutDataTypeStr=Inherit: Same as first input
  Product1 : Product  Inputs=3  SaturateOnIntegerOverflow=on  OutDataTypeStr=Inherit: Same as first input
  Product2 : Product  SaturateOnIntegerOverflow=on  OutDataTypeStr=Inherit: Same as first input
  Rd : Gain  Gain=R  SaturateOnIntegerOverflow=on  OutDataTypeStr=Inherit: Same as input  ParamDataTypeStr=Inherit: Same as input
  Rq : Gain  Gain=R  SaturateOnIntegerOverflow=on  OutDataTypeStr=Inherit: Same as input  ParamDataTypeStr=Inherit: Same as input
  Sum : Sum  Inputs=|++  SaturateOnIntegerOverflow=on
  Sum1 : Sum  Inputs=|+-+  SaturateOnIntegerOverflow=on
  Sum2 : Sum  Inputs=|+---  SaturateOnIntegerOverflow=on
  initial angel : Step  Time=0  After=13*pi/9  SampleTime=0
  sqrt(3) : Gain  Gain=sqrt(3)  SaturateOnIntegerOverflow=on  OutDataTypeStr=Inherit: Same as input  ParamDataTypeStr=Inherit: Same as input
  id : Outport
  iq : Outport  Port=2
  phase : Outport  Port=3
  u : Outport  Port=4
  tag scope: phase=global
  wires:
  Sum/1 -> Mux/7, phase/1, [phase]
  Integrator/1 -> Sum/1
  initial angel/1 -> Sum/2
  w/1 -> Product2/2, Integrator/1, Product1/3, Product/3
  Mux/1 -> Fcn/1, Fcn1/1, u/1
  Fcn/1 -> Sum1/1
  Sum1/1 -> 1/Ld/1
  1/Ld/1 -> Integrator1/1
  Integrator1/1 -> Rd/1, id/1, Product1/2
  Rd/1 -> Sum1/2
  Fcn1/1 -> Sum2/1
  Sum2/1 -> 1/Lq/1
  1/Lq/1 -> Integrator2/1
  Integrator2/1 -> Rq/1, iq/1, Product/2
  Rq/1 -> Sum2/2
  Product/1 -> Sum1/3
  Product1/1 -> Sum2/3
  Product2/1 -> sqrt(3)/1
  psi/1 -> Product2/1
  Lq/1 -> Product/1
  Ld/1 -> Product1/1
  ud/1 -> Mux/1
  ua/1 -> Mux/2
  ue/1 -> Mux/3
  ub/1 -> Mux/4
  uf/1 -> Mux/5
  uc/1 -> Mux/6
  sqrt(3)/1 -> Sum2/4

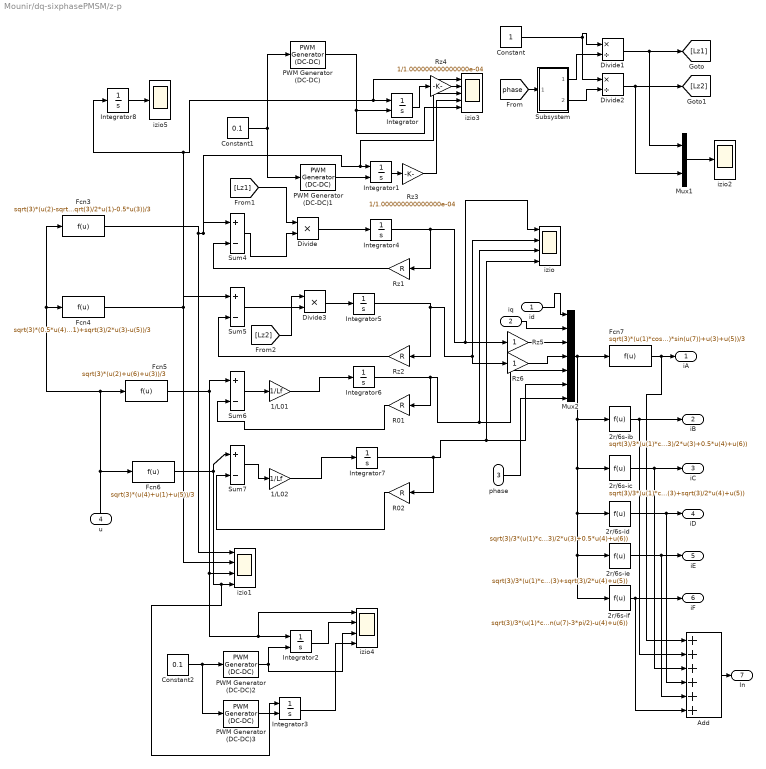
== system Mounir/dq-sixphasePMSM/z-p ==
  id : Inport
  iq : Inport  Port=2
  phase : Inport  Port=3
  u : Inport  Port=4
  1/L01 : Gain  Gain=1/Lf  SaturateOnIntegerOverflow=on  OutDataTypeStr=Inherit: Same as input  ParamDataTypeStr=Inherit: Same as input
  1/L02 : Gain  Gain=1/Lf  SaturateOnIntegerOverflow=on  OutDataTypeStr=Inherit: Same as input  ParamDataTypeStr=Inherit: Same as input
  2r/6s-ib : Fcn  Expr=sqrt(3)/3*(u(1)*cos(u(7)-pi/6)-u(2)*sin(u(7)-pi/6)-sqrt(3)/2*u(3)+0.5*u(4)+u(6))
  2r/6s-ic : Fcn  Expr=sqrt(3)/3*(u(1)*cos(u(7)-2*pi/3)-u(2)*sin(u(7)-2*pi/3)-0.5*u(3)+sqrt(3)/2*u(4)+u(5))
  2r/6s-id : Fcn  Expr=sqrt(3)/3*(u(1)*cos(u(7)-5*pi/6)-u(2)*sin(u(7)-5*pi/6)+sqrt(3)/2*u(3)+0.5*u(4)+u(6))
  2r/6s-ie : Fcn  Expr=sqrt(3)/3*(u(1)*cos(u(7)-4*pi/3)-u(2)*sin(u(7)-4*pi/3)-0.5*u(3)+sqrt(3)/2*u(4)+u(5))
  2r/6s-if : Fcn  Expr=sqrt(3)/3*(u(1)*cos(u(7)-3*pi/2)-u(2)*sin(u(7)-3*pi/2)-u(4)+u(6))
  Add : Sum  Inputs=++++++
  Constant : Constant
  Constant1 : Constant  Value=0.1
  Constant2 : Constant  Value=0.1
  Divide : Product  Inputs=**
  Divide1 : Product  Inputs=*/
  Divide2 : Product  Inputs=*/
  Divide3 : Product  Inputs=**
  Fcn3 : Fcn  Expr=sqrt(3)*(u(2)-sqrt(3)/2*u(4)-0.5*u(6)+sqrt(3)/2*u(1)-0.5*u(3))/3
  Fcn4 : Fcn  Expr=sqrt(3)*(0.5*u(4)-sqrt(3)/2*u(6)+0.5*u(1)+sqrt(3)/2*u(3)-u(5))/3
  Fcn5 : Fcn  Expr=sqrt(3)*(u(2)+u(6)+u(3))/3
  Fcn6 : Fcn  Expr=sqrt(3)*(u(4)+u(1)+u(5))/3
  Fcn7 : Fcn  Expr=sqrt(3)*(u(1)*cos(u(7))-u(2)*sin(u(7))+u(3)+u(5))/3
  Integrator{,1..3} (4 alike) : Integrator  ExternalReset=rising
  Integrator{4..8} (5 alike) : Integrator
  Mux1 : Mux  Inputs=2
  Mux2 : Mux  Inputs=7
  PWM Generator (DC-DC){,1..3} (4 alike) : powerlib_meascontrol/Pulse & Signal Generators/PWM Generator (DC-DC)  Fsw=1/1.000000000000000e-04  Ts=0
  R01 : Gain  Gain=R  SaturateOnIntegerOverflow=on  OutDataTypeStr=Inherit: Same as input  ParamDataTypeStr=Inherit: Same as input
  R02 : Gain  Gain=R  SaturateOnIntegerOverflow=on  OutDataTypeStr=Inherit: Same as input  ParamDataTypeStr=Inherit: Same as input
  Rz1 : Gain  Gain=R  SaturateOnIntegerOverflow=on  OutDataTypeStr=Inherit: Same as input  ParamDataTypeStr=Inherit: Same as input
  Rz2 : Gain  Gain=R  SaturateOnIntegerOverflow=on  OutDataTypeStr=Inherit: Same as input  ParamDataTypeStr=Inherit: Same as input
  Rz3 : Gain  Gain=1/1.000000000000000e-04  SaturateOnIntegerOverflow=on  OutDataTypeStr=Inherit: Same as input  ParamDataTypeStr=Inherit: Same as input
  Rz4 : Gain  Gain=1/1.000000000000000e-04  SaturateOnIntegerOverflow=on  OutDataTypeStr=Inherit: Same as input  ParamDataTypeStr=Inherit: Same as input
  Rz5 : Gain  SaturateOnIntegerOverflow=on  OutDataTypeStr=Inherit: Same as input  ParamDataTypeStr=Inherit: Same as input
  Rz6 : Gain  SaturateOnIntegerOverflow=on  OutDataTypeStr=Inherit: Same as input  ParamDataTypeStr=Inherit: Same as input
  Subsystem : Subsystem
  Sum{4..7} (4 alike) : Sum  Inputs=|+-  SaturateOnIntegerOverflow=on
  izio : Scope  NumInputPorts=4
      settings: TimeRange=0.25  YMin=-4~-4~-1.25e-15~-1.25e-15  YMax=2.5~4~1.25e-15~1.25e-15  SaveName=ScopeData9
  izio1 : Scope  NumInputPorts=4
      settings: TimeRange=0.25  YMin=-200~-200~-4e-14~-4e-14  YMax=200~200~4e-14~4e-14  SaveName=ScopeData11
  izio2 : Scope
      settings: TimeRange=0.25  YMin=1761.2  YMax=1761.6  SaveName=ScopeData18
  izio3 : Scope  NumInputPorts=5
      settings: TimeRange=0.25  YMin=-150~-30~-150~-30~0  YMax=150~40~150~40~1  SaveName=ScopeData19
  izio4 : Scope  NumInputPorts=4
      settings: TimeRange=0.25  YMin=-4e-14~-7.5e-19~0~-1e-18  YMax=4e-14~1e-18~1~1e-18  SaveName=ScopeData20
  izio5 : Scope
      settings: TimeRange=0.25  YMin=1761.2  YMax=1761.6  SaveName=ScopeData8
  iA : Outport
  iB : Outport  Port=2
  iC : Outport  Port=3
  iD : Outport  Port=4
  iE : Outport  Port=5
  iF : Outport  Port=6
  In : Outport  Port=7
  wires:
  Mux2/1 -> Fcn7/1, 2r/6s-ic/1, 2r/6s-id/1, 2r/6s-ie/1, 2r/6s-if/1, 2r/6s-ib/1
  R02/1 -> Sum7/2
  R01/1 -> Sum6/2
  Rz2/1 -> Sum5/2
  Rz1/1 -> Sum4/2
  Integrator7/1 -> R02/1, Mux2/6, izio/4
  1/L02/1 -> Integrator7/1
  Sum7/1 -> 1/L02/1
  Integrator6/1 -> R01/1, Mux2/5, izio/3
  1/L01/1 -> Integrator6/1
  Sum6/1 -> 1/L01/1
  id/1 -> Mux2/1
  iq/1 -> Mux2/2
  u/1 -> Fcn4/1, Fcn3/1, Fcn5/1, Fcn6/1
  phase/1 -> Mux2/7
  Fcn7/1 -> Add/1, iA/1
  2r/6s-ib/1 -> Add/2, iB/1
  2r/6s-id/1 -> Add/4, iD/1
  2r/6s-ie/1 -> Add/5, iE/1
  2r/6s-if/1 -> Add/6, iF/1
  [phase] -> Subsystem/1(Phase)
  Subsystem/1(Lz1) -> Divide1/2
  Divide1/1 -> Mux1/1, [Lz1]
  Constant/1 -> Divide1/1, Divide2/1
  Subsystem/2(Lz2) -> Divide2/2
  Divide2/1 -> Mux1/2, [Lz2]
  Mux1/1 -> izio2/1
  Sum4/1 -> Divide/2
  [Lz1] -> Divide/1
  Divide/1 -> Integrator4/1
  Divide3/1 -> Integrator5/1
  Sum5/1 -> Divide3/2
  [Lz2] -> Divide3/1
  Constant1/1 -> PWM Generator (DC-DC)/1, PWM Generator (DC-DC)1/1
  PWM Generator (DC-DC)/1 -> izio3/5, Integrator/2
  PWM Generator (DC-DC)1/1 -> Integrator1/2
  Fcn6/1 -> Sum7/1, Integrator3/1, izio1/4
  Fcn5/1 -> Sum6/1, izio4/1, Integrator2/1, izio1/3
  Constant2/1 -> PWM Generator (DC-DC)3/1, PWM Generator (DC-DC)2/1
  PWM Generator (DC-DC)2/1 -> Integrator2/2, izio4/3
  Integrator2/1 -> izio4/2
  PWM Generator (DC-DC)3/1 -> Integrator3/2
  Integrator3/1 -> izio4/4
  Integrator1/1 -> Rz3/1
  Rz3/1 -> izio3/4
  Integrator5/1 -> Rz2/1, Rz6/1, izio/2
  Rz4/1 -> izio3/2
  Integrator/1 -> Rz4/1
  Integrator4/1 -> Rz1/1, Rz5/1, izio/1
  Rz5/1 -> Mux2/3
  Rz6/1 -> Mux2/4
  Integrator8/1 -> izio5/1
  Fcn3/1 -> izio1/1, izio3/3, Integrator1/1, Sum4/1
  Fcn4/1 -> Sum5/1, izio3/1, Integrator/1, Integrator8/1, izio1/2
  Add/1 -> In/1
  2r/6s-ic/1 -> Add/3, iC/1

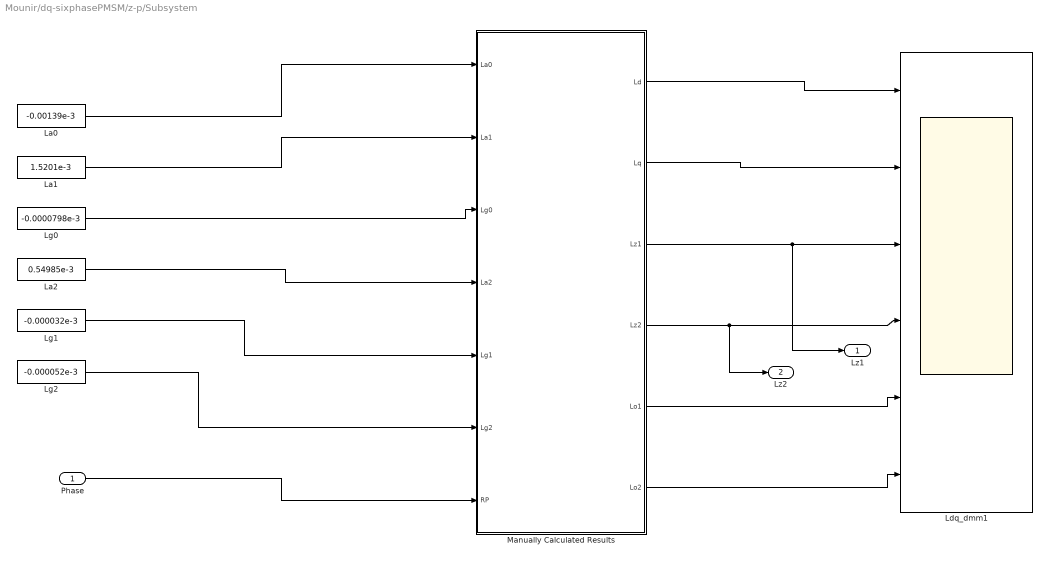
== system Mounir/dq-sixphasePMSM/z-p/Subsystem ==
  Phase : Inport
  La0 : Constant  Value=-0.00139e-3
  La1 : Constant  Value=1.5201e-3
  La2 : Constant  Value=0.54985e-3
  Ldq_dmm1 : Scope  NumInputPorts=6
      settings: YMin=0.00234476~0.002345~0.00056767~0.00056767~0.00144409~0.00144409  YMax=0.00259158~0.00259184~0.0005678~0.0005678~0.00159611~0.00159611  SaveName=ScopeData25
  Lg0 : Constant  Value=-0.0000798e-3
  Lg1 : Constant  Value=-0.000032e-3
  Lg2 : Constant  Value=-0.000052e-3
  "Manually Calculated Results " : MATLAB Function  TreatAsAtomicUnit=on
  Lz1 : Outport
  Lz2 : Outport  Port=2
  wires:
  "Manually Calculated Results "/3(Lz1) -> Lz1/1, Ldq_dmm1/3
  Lg2/1 -> "Manually Calculated Results "/6(Lg2)
  Lg1/1 -> "Manually Calculated Results "/5(Lg1)
  "Manually Calculated Results "/2(Lq) -> Ldq_dmm1/2
  Lg0/1 -> "Manually Calculated Results "/3(Lg0)
  "Manually Calculated Results "/4(Lz2) -> Lz2/1, Ldq_dmm1/4
  "Manually Calculated Results "/6(Lo2) -> Ldq_dmm1/6
  "Manually Calculated Results "/1(Ld) -> Ldq_dmm1/1
  "Manually Calculated Results "/5(Lo1) -> Ldq_dmm1/5
  La0/1 -> "Manually Calculated Results "/1(La0)
  La1/1 -> "Manually Calculated Results "/2(La1)
  La2/1 -> "Manually Calculated Results "/4(La2)
  Phase/1 -> "Manually Calculated Results "/7(RP)

== matlab function Mounir/inverter_phase_voltages_matrix ==
  data: uo output; uab input; ua output; ubc input; ucd input; ude input; uef input; ub output; uc output; ud output; ue output; uf output
function [uo,ua,ub,uc,ud,ue,uf] = fcn(uab,ubc,ucd,ude,uef)

%#eml
uxx=[uab,ubc,ucd,ude,uef,0,0]';
T=1/6*[2 0 2 0 2 -2 2;
4 4 2 2 0 2 0;
0 4 4 2 2 0 2;
-2 -2 2 2 0 2 0;
0 -2 -2 2 2 0 2;
-2 -2 -4 -4 0 2 0;
0 -2 -2 -4 -4 0 2];
I=T*uxx;
uo=I(1);
ua=I(2);
ub=I(3);
uc=I(4);
ud=I(5);
ue=I(6);
uf=I(7);

== matlab function Mounir/inverter -phase-voltage_matrix  ==
  data: uo output; uab input; ua output; ubc input; ucd input; ude input; uef input; ub output; uc output; ud output; ue output; uf output
function [uo,ua,ub,uc,ud,ue,uf] = fcn(uab,ubc,ucd,ude,uef)

%#eml
uxx=[uab,ubc,ucd,ude,uef,0,0]';
T=1/6*[2 0 2 0 2 -2 2;
4 4 2 2 0 2 0;
0 4 4 2 2 0 2;
-2 -2 2 2 0 2 0;
0 -2 -2 2 2 0 2;
-2 -2 -4 -4 0 2 0;
0 -2 -2 -4 -4 0 2];
I=T*uxx;
uo=I(1);
ua=I(2);
ub=I(3);
uc=I(4);
ud=I(5);
ue=I(6);
uf=I(7);

== matlab function Mounir/SVPWM2/Embedded MATLAB Function6 ==
  data: N output; ualfa input; ubeta input; R output
function [N,R] = fcn(ualfa,ubeta)

%#xsxx
[TH,R] = cart2pol(ualfa,ubeta);
if TH<0
    TH=TH+2*pi;
end
N=floor((TH+pi/12)/(pi/6))+1;
if N==13
    N=1;
end;
%N=floor((TH)/(pi/3))+1;

== matlab function Mounir/SVPWM2/Embedded MATLAB Function7 ==
  data: N input; T1 output; ualfa input; ubeta input; Tpwm input; T2 output; T3 output; T4 output; T0 output; udc input
function [T1,T2,T3,T4,T0] = fcn(N,ualfa,ubeta,Tpwm,udc)
u=udc*sqrt(3)*[0.455341801	-0.455341801	-0.122008468	0.122008468;
0.622008468	-0.166666667	0.044658199	-0.166666667;
0.622008468	0.166666667	0.044658199	0.166666667;
0.455341801	0.455341801	-0.122008468	-0.122008468;
0.166666667	0.622008468	0.166666667	0.044658199;
-0.166666667	0.622008468	-0.166666667	0.044658199;
-0.455341801	0.455341801	0.122008468	-0.122008468;
-0.622008468	0.166666667	-0.044658199	0.166666667;
-0.622008468	-0.166666667	-0.044658199	-0.166666667;
-0.455341801	-0.455341801	0.122008468	0.122008468;
-0.166666667	-0.622008468	-0.166666667	-0.044658199;
0.166666667	-0.622008468	0.166666667	-0.044658199;
0.455341801	-0.455341801	-0.122008468	0.122008468;
0.622008468	-0.166666667	0.044658199	-0.166666667;
0.622008468	0.166666667	0.044658199	0.166666667];
A=[u(N,1) u(N+1,1) u(N+2,1) u(N+3,1);
u(N,2) u(N+1,2) u(N+2,2) u(N+3,2);
u(N,3) u(N+1,3) u(N+2,3) u(N+3,3);
u(N,4) u(N+1,4) u(N+2,4) u(N+3,4)];
b=[ualfa*Tpwm;ubeta*Tpwm;0;0];
T=inv(A)*b;
T1=T(1);
T2=T(2);
T3=T(3);
T4=T(4);
Tsum=T1+T2+T3+T4;
if Tsum>Tpwm
    T1=T1*Tpwm/Tsum;
    T2=T2*Tpwm/Tsum;
    T3=T3*Tpwm/Tsum;
    T4=T4*Tpwm/Tsum;
end
T0=Tpwm-T1-T2-T3-T4;

== matlab function Mounir/SVPWM2/rest of others ==
  data: N input; T1 input; T2 input; T3 input; T4 input; T0 input; Tcma1 output; Tcma2 output; Tcmb1 output; Tcmb2 output; Tcmc1 output; Tcmc2 output; Tcmd1 output; Tcmd2 output; Tcme1 output; Tcme2 output; Tcmf1 output; Tcmf2 output
function [Tcma1,Tcma2,Tcmb1,Tcmb2,Tcmc1,Tcmc2,Tcmd1,Tcmd2,Tcme1,Tcme2,Tcmf1,Tcmf2] = fcn(N,T1,T2,T3,T4,T0)

%#xsxx
Ta=T0/4;
Tb=Ta+T2;
Tc=Tb+T1;
Td=Tc+T0/2;
Te=Td+T4;
Tf=Te+T3;
Td=Td;
Te=Te;
Tf=Tf;
Ta1=T0/4;
Tb1=Ta1+T1;
Tc1=Tb1+T2;
Td1=Tc1+T0/2;
Te1=Td1+T3;
Tf1=Te1+T4;
Td1=Td1;
Te1=Te1;
Tf1=Tf1;
    Tcma1=0;
    Tcma2=0;
    Tcmb1=0;
    Tcmb2=0;
    Tcmc1=0;
    Tcmc2=0;
    Tcmd1=0;
    Tcmd2=0;
    Tcme1=0;
    Tcme2=0;
    Tcmf1=0;
    Tcmf2=0;
if N==1
    Tcma1=Ta;%TIme of "00" voltage vector 
    Tcma2=Tf;%TIme of "48" voltage vector 
    Tcmb1=Ta;
    Tcmb2=Tf;
    Tcmc1=Tc;%TIme of "51" voltage vector 
    Tcmc2=Te;%TIme of "56" voltage vector 
    Tcmd1=Tc;
    Tcmd2=Td;
    Tcme1=Tb;%TIme of "49" voltage vector 
    Tcme2=Td;%TIme of "63" voltage vector 
    Tcmf1=Ta;
    Tcmf2=Td;
end
if N==2
    Tcma1=Ta;
    Tcma2=Tf;
    Tcmb1=Ta;
    Tcmb2=Tf;
    Tcmc1=Tc;
    Tcmc2=Tf;
    Tcmd1=Tc;
    Tcmd2=Te;
    Tcme1=Tc;
    Tcme2=Td;
    Tcmf1=Tb;
    Tcmf2=Td;
end
if N==3
    Tcma1=Ta1;
    Tcma2=Te1;
    Tcmb1=Ta1;
    Tcmb2=Tf1;
    Tcmc1=Tb1;
    Tcmc2=Tf1;
    Tcmd1=Tc1;
    Tcmd2=Tf1;
    Tcme1=Tc1;
    Tcme2=Td1;
    Tcmf1=Tc1;
    Tcmf2=Td1;
end
if N==4
    Tcma1=Ta1;
    Tcma2=Td1;
    Tcmb1=Ta1;
    Tcmb2=Te1;
    Tcmc1=Ta1;
    Tcmc2=Tf1;
    Tcmd1=Tb1;
    Tcmd2=Tf1;
    Tcme1=Tc1;
    Tcme2=Td1;
    Tcmf1=Tc1;
    Tcmf2=Td1;
end
if N==5
    Tcma1=Tb;
    Tcma2=Td;
    Tcmb1=Ta;
    Tcmb2=Td;
    Tcmc1=Ta;
    Tcmc2=Tf;
    Tcmd1=Ta;
    Tcmd2=Tf;
    Tcme1=Tc;
    Tcme2=Te;
    Tcmf1=Tc;
    Tcmf2=Td;
end
if N==6
    Tcma1=Tc;
    Tcma2=Td;
    Tcmb1=Tb;
    Tcmb2=Td;
    Tcmc1=Ta;
    Tcmc2=Tf;
    Tcmd1=Ta;
    Tcmd2=Tf;
    Tcme1=Tc;
    Tcme2=Tf;
    Tcmf1=Tc;
    Tcmf2=Te;
end
if N==7
    Tcma1=Tc1;
    Tcma2=Td1;
    Tcmb1=Tc1;
    Tcmb2=Td1;
    Tcmc1=Ta1;
    Tcmc2=Te1;
    Tcmd1=Ta1;
    Tcmd2=Tf1;
    Tcme1=Tb1;
    Tcme2=Tf1;
    Tcmf1=Tc1;
    Tcmf2=Tf1;
end
if N==8
    Tcma1=Tc1;
    Tcma2=Td1;
    Tcmb1=Tc1;
    Tcmb2=Td1;
    Tcmc1=Ta1;
    Tcmc2=Td1;
    Tcmd1=Ta1;
    Tcmd2=Te1;
    Tcme1=Ta1;
    Tcme2=Tf1;
    Tcmf1=Tb1;
    Tcmf2=Tf1;
end
if N==9
    Tcma1=Tc;
    Tcma2=Te;
    Tcmb1=Tc;
    Tcmb2=Td;
    Tcmc1=Tb;
    Tcmc2=Td;
    Tcmd1=Ta;
    Tcmd2=Td;
    Tcme1=Ta;
    Tcme2=Tf;
    Tcmf1=Ta;
    Tcmf2=Tf;
end
if N==10
    Tcma1=Tc;
    Tcma2=Tf;
    Tcmb1=Tc;
    Tcmb2=Te;
    Tcmc1=Tc;
    Tcmc2=Td;
    Tcmd1=Tb;
    Tcmd2=Td;
    Tcme1=Ta;
    Tcme2=Tf;
    Tcmf1=Ta;
    Tcmf2=Tf;
end
if N==11
    Tcma1=Tb1;
    Tcma2=Tf1;
    Tcmb1=Tc1;
    Tcmb2=Tf1;
    Tcmc1=Tc1;
    Tcmc2=Td1;
    Tcmd1=Tc1;
    Tcmd2=Td1;
    Tcme1=Ta1;
    Tcme2=Te1;
    Tcmf1=Ta1;
    Tcmf2=Tf1;
end
if N==12
    Tcma1=Ta1;
    Tcma2=Tf1;
    Tcmb1=Tb1;
    Tcmb2=Tf1;
    Tcmc1=Tc1;
    Tcmc2=Td1;
    Tcmd1=Tc1;
    Tcmd2=Td1;
    Tcme1=Ta1;
    Tcme2=Td1;
    Tcmf1=Ta1;
    Tcmf2=Te1;
end

== matlab function Mounir/dq-sixphasePMSM/z-p/Subsystem/Manually Calculated Results  ==
  data: La0 input; Ld output; La1 input; Lg0 input; La2 input; Lg1 input; Lg2 input; RP input; Lq output; Lz1 output; Lz2 output; Lo1 output; Lo2 output
function [Ld,Lq,Lz1,Lz2,Lo1,Lo2] = fcn(La0,La1,Lg0,La2,Lg1,Lg2,RP)
%#codegen
Ld=3*La0+La1+sqrt(3)*La2+(1/2*Lg0+Lg1+Lg2);
Lq=3*La0+sqrt(3)*La2+La1-(1/2*Lg0+Lg1+Lg2);
Lz1=La1+cos(2*RP)*(1/2*Lg0-Lg1+Lg2)-sqrt(3)*La2;
Lz2=La1-cos(2*RP)*(1/2*Lg0-Lg1+Lg2)-sqrt(3)*La2;
Lo1=La1;
Lo2=La1;

== matlab function Mounir/SVPWM1/Embedded MATLAB Function6 ==
  data: N output; ualfa input; ubeta input; R output
function [N,R] = fcn(ualfa,ubeta)

%#xsxx
[TH,R] = cart2pol(ualfa,ubeta);
if TH<0
    TH=TH+2*pi;
end
N=floor((TH+pi/12)/(pi/6))+1;
if N==13
    N=1;
end;
%N=floor((TH)/(pi/3))+1;

== matlab function Mounir/SVPWM1/Embedded MATLAB Function7 ==
  data: N input; T1 output; ualfa input; ubeta input; Tpwm input; T2 output; T3 output; T4 output; T0 output; udc input
function [T1,T2,T3,T4,T0] = fcn(N,ualfa,ubeta,Tpwm,udc)
u=udc*sqrt(3)*[0.455341801	-0.455341801	-0.122008468	0.122008468;
0.622008468	-0.166666667	0.044658199	-0.166666667;
0.622008468	0.166666667	0.044658199	0.166666667;
0.455341801	0.455341801	-0.122008468	-0.122008468;
0.166666667	0.622008468	0.166666667	0.044658199;
-0.166666667	0.622008468	-0.166666667	0.044658199;
-0.455341801	0.455341801	0.122008468	-0.122008468;
-0.622008468	0.166666667	-0.044658199	0.166666667;
-0.622008468	-0.166666667	-0.044658199	-0.166666667;
-0.455341801	-0.455341801	0.122008468	0.122008468;
-0.166666667	-0.622008468	-0.166666667	-0.044658199;
0.166666667	-0.622008468	0.166666667	-0.044658199;
0.455341801	-0.455341801	-0.122008468	0.122008468;
0.622008468	-0.166666667	0.044658199	-0.166666667;
0.622008468	0.166666667	0.044658199	0.166666667];
A=[u(N,1) u(N+1,1) u(N+2,1) u(N+3,1);
u(N,2) u(N+1,2) u(N+2,2) u(N+3,2);
u(N,3) u(N+1,3) u(N+2,3) u(N+3,3);
u(N,4) u(N+1,4) u(N+2,4) u(N+3,4)];
b=[ualfa*Tpwm;ubeta*Tpwm;0;0];
T=inv(A)*b;
T1=T(1);
T2=T(2);
T3=T(3);
T4=T(4);
Tsum=T1+T2+T3+T4;
if Tsum>Tpwm
    T1=T1*Tpwm/Tsum;
    T2=T2*Tpwm/Tsum;
    T3=T3*Tpwm/Tsum;
    T4=T4*Tpwm/Tsum;
end
T0=Tpwm-T1-T2-T3-T4;

== matlab function Mounir/SVPWM1/rest of others ==
  data: N input; T1 input; T2 input; T3 input; T4 input; T0 input; Tcma1 output; Tcma2 output; Tcmb1 output; Tcmb2 output; Tcmc1 output; Tcmc2 output; Tcmd1 output; Tcmd2 output; Tcme1 output; Tcme2 output; Tcmf1 output; Tcmf2 output
function [Tcma1,Tcma2,Tcmb1,Tcmb2,Tcmc1,Tcmc2,Tcmd1,Tcmd2,Tcme1,Tcme2,Tcmf1,Tcmf2] = fcn(N,T1,T2,T3,T4,T0)

%#xsxx
Ta=T0/4;
Tb=Ta+T2;
Tc=Tb+T1;
Td=Tc+T0/2;
Te=Td+T4;
Tf=Te+T3;
Td=Td;
Te=Te;
Tf=Tf;
Ta1=T0/4;
Tb1=Ta1+T1;
Tc1=Tb1+T2;
Td1=Tc1+T0/2;
Te1=Td1+T3;
Tf1=Te1+T4;
Td1=Td1;
Te1=Te1;
Tf1=Tf1;
    Tcma1=0;
    Tcma2=0;
    Tcmb1=0;
    Tcmb2=0;
    Tcmc1=0;
    Tcmc2=0;
    Tcmd1=0;
    Tcmd2=0;
    Tcme1=0;
    Tcme2=0;
    Tcmf1=0;
    Tcmf2=0;
if N==1
    Tcma1=Ta;%TIme of "00" voltage vector 
    Tcma2=Tf;%TIme of "48" voltage vector 
    Tcmb1=Ta;
    Tcmb2=Tf;
    Tcmc1=Tc;%TIme of "51" voltage vector 
    Tcmc2=Te;%TIme of "56" voltage vector 
    Tcmd1=Tc;
    Tcmd2=Td;
    Tcme1=Tb;%TIme of "49" voltage vector 
    Tcme2=Td;%TIme of "63" voltage vector 
    Tcmf1=Ta;
    Tcmf2=Td;
end
if N==2
    Tcma1=Ta;
    Tcma2=Tf;
    Tcmb1=Ta;
    Tcmb2=Tf;
    Tcmc1=Tc;
    Tcmc2=Tf;
    Tcmd1=Tc;
    Tcmd2=Te;
    Tcme1=Tc;
    Tcme2=Td;
    Tcmf1=Tb;
    Tcmf2=Td;
end
if N==3
    Tcma1=Ta1;
    Tcma2=Te1;
    Tcmb1=Ta1;
    Tcmb2=Tf1;
    Tcmc1=Tb1;
    Tcmc2=Tf1;
    Tcmd1=Tc1;
    Tcmd2=Tf1;
    Tcme1=Tc1;
    Tcme2=Td1;
    Tcmf1=Tc1;
    Tcmf2=Td1;
end
if N==4
    Tcma1=Ta1;
    Tcma2=Td1;
    Tcmb1=Ta1;
    Tcmb2=Te1;
    Tcmc1=Ta1;
    Tcmc2=Tf1;
    Tcmd1=Tb1;
    Tcmd2=Tf1;
    Tcme1=Tc1;
    Tcme2=Td1;
    Tcmf1=Tc1;
    Tcmf2=Td1;
end
if N==5
    Tcma1=Tb;
    Tcma2=Td;
    Tcmb1=Ta;
    Tcmb2=Td;
    Tcmc1=Ta;
    Tcmc2=Tf;
    Tcmd1=Ta;
    Tcmd2=Tf;
    Tcme1=Tc;
    Tcme2=Te;
    Tcmf1=Tc;
    Tcmf2=Td;
end
if N==6
    Tcma1=Tc;
    Tcma2=Td;
    Tcmb1=Tb;
    Tcmb2=Td;
    Tcmc1=Ta;
    Tcmc2=Tf;
    Tcmd1=Ta;
    Tcmd2=Tf;
    Tcme1=Tc;
    Tcme2=Tf;
    Tcmf1=Tc;
    Tcmf2=Te;
end
if N==7
    Tcma1=Tc1;
    Tcma2=Td1;
    Tcmb1=Tc1;
    Tcmb2=Td1;
    Tcmc1=Ta1;
    Tcmc2=Te1;
    Tcmd1=Ta1;
    Tcmd2=Tf1;
    Tcme1=Tb1;
    Tcme2=Tf1;
    Tcmf1=Tc1;
    Tcmf2=Tf1;
end
if N==8
    Tcma1=Tc1;
    Tcma2=Td1;
    Tcmb1=Tc1;
    Tcmb2=Td1;
    Tcmc1=Ta1;
    Tcmc2=Td1;
    Tcmd1=Ta1;
    Tcmd2=Te1;
    Tcme1=Ta1;
    Tcme2=Tf1;
    Tcmf1=Tb1;
    Tcmf2=Tf1;
end
if N==9
    Tcma1=Tc;
    Tcma2=Te;
    Tcmb1=Tc;
    Tcmb2=Td;
    Tcmc1=Tb;
    Tcmc2=Td;
    Tcmd1=Ta;
    Tcmd2=Td;
    Tcme1=Ta;
    Tcme2=Tf;
    Tcmf1=Ta;
    Tcmf2=Tf;
end
if N==10
    Tcma1=Tc;
    Tcma2=Tf;
    Tcmb1=Tc;
    Tcmb2=Te;
    Tcmc1=Tc;
    Tcmc2=Td;
    Tcmd1=Tb;
    Tcmd2=Td;
    Tcme1=Ta;
    Tcme2=Tf;
    Tcmf1=Ta;
    Tcmf2=Tf;
end
if N==11
    Tcma1=Tb1;
    Tcma2=Tf1;
    Tcmb1=Tc1;
    Tcmb2=Tf1;
    Tcmc1=Tc1;
    Tcmc2=Td1;
    Tcmd1=Tc1;
    Tcmd2=Td1;
    Tcme1=Ta1;
    Tcme2=Te1;
    Tcmf1=Ta1;
    Tcmf2=Tf1;
end
if N==12
    Tcma1=Ta1;
    Tcma2=Tf1;
    Tcmb1=Tb1;
    Tcmb2=Tf1;
    Tcmc1=Tc1;
    Tcmc2=Td1;
    Tcmd1=Tc1;
    Tcmd2=Td1;
    Tcme1=Ta1;
    Tcme2=Td1;
    Tcmf1=Ta1;
    Tcmf2=Te1;
end
